simulink model "Lecture7Exercise"  (R2020b)
settings: Solver=VariableStepAuto  StartTime=0.0  StopTime=10.0  RelTol=1e-3
values from neighbouring files (symbols this model uses):
  A = [-Ra/La -Ka/La; Ka/J -B/J]    [Lecture10_11Exercise.m]    (also in Lecture5Exercises.m = [2.7 0.8 0.7; 1 0 0; 0 1 0]; Lecture6Exercise.m = [0 1 0; 0 -B/J Ka/J; 0 -Km/La -Ra/La]; Lecture7Exercise.m = [0, 1; -1, -2])
  B = [1/La;0]    [Lecture10_11Exercise.m]    (also in Lecture5Exercises.m = [1; 0; 0]; Lecture6Exercise.m = [0; 0; 1/La]; Lecture7Exercise.m = [0; 1])
  B1 = [1; 1]    [Lecture7Exercise.m]
  C = [0 1]    [Lecture10_11Exercise.m]    (also in Lecture5Exercises.m = [0 0 1]; Lecture6Exercise.m = [1 0 0]; Lecture7Exercise.m = [1, 0])
  K = [KKi(1) KKi(2)]    [Lecture4Exercise.m]    (also in Lecture5Exercises.m = acker(A_adj, B_adj, [z_p z_p z_p]); Lecture9Exercise.m = P\D)
  L = 1    [Lecture1Pendulum.m]    (also in Lecture5Exercises.m = acker(A_bb', A_ab', [zper zper])')
  Rv = 1    [Lecture7Exercise.m]
  Rw = 1    [Lecture7Exercise.m]
settings Model: Creator=sebastian  LastModifiedBy=sebastian

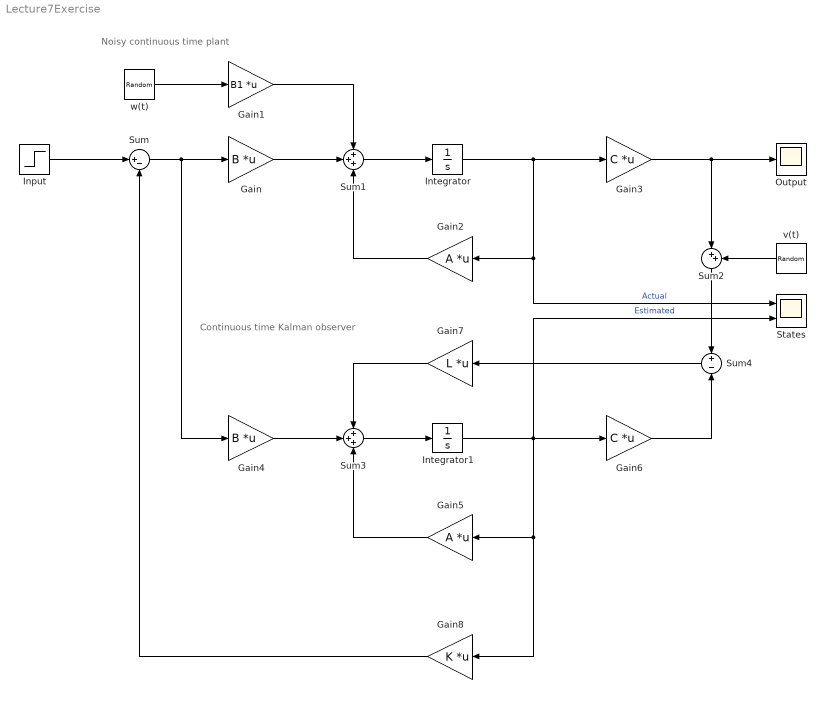
== system Lecture7Exercise ==
  note: Continuous time Kalman observer
  note: Noisy continuous time plant
  Gain : Gain  Gain=B  Multiplication=Matrix(K*u)
  Gain1 : Gain  Gain=B1  Multiplication=Matrix(K*u)
  Gain2 : Gain  Gain=A  Multiplication=Matrix(K*u)
  Gain3 : Gain  Gain=C  Multiplication=Matrix(K*u)
  Gain4 : Gain  Gain=B  Multiplication=Matrix(K*u)
  Gain5 : Gain  Gain=A  Multiplication=Matrix(K*u)
  Gain6 : Gain  Gain=C  Multiplication=Matrix(K*u)
  Gain7 : Gain  Gain=L  Multiplication=Matrix(K*u)
  Gain8 : Gain  Gain=K  Multiplication=Matrix(K*u)
  Input : Step  SampleTime=0
  Integrator : Integrator
  Integrator1 : Integrator
  Output : Scope
  States : Scope  NumInputPorts=2
  Sum : Sum  Inputs=|+-
  Sum1 : Sum  Inputs=+++
  Sum2 : Sum  Inputs=|++
  Sum3 : Sum  Inputs=+++
  Sum4 : Sum  Inputs=+-
  v(t) : RandomNumber  Variance=Rv  SampleTime=0.01
  w(t) : RandomNumber  Variance=Rw  SampleTime=0.01
  wires:
  Sum/1 -> Gain4/1, Gain/1
  Gain/1 -> Sum1/2
  Gain1/1 -> Sum1/1
  w(t)/1 -> Gain1/1
  Sum1/1 -> Integrator/1
  Integrator/1 -> Gain3/1, States/1, Gain2/1  "Actual"
  Gain2/1 -> Sum1/3
  Gain3/1 -> Sum2/1, Output/1
  v(t)/1 -> Sum2/2
  Input/1 -> Sum/1
  Gain4/1 -> Sum3/2
  Gain5/1 -> Sum3/3
  Integrator1/1 -> States/2, Gain6/1, Gain8/1, Gain5/1  "Estimated"
  Sum3/1 -> Integrator1/1
  Sum4/1 -> Gain7/1
  Sum2/1 -> Sum4/1
  Gain6/1 -> Sum4/2
  Gain7/1 -> Sum3/1
  Gain8/1 -> Sum/2
